simulink model "LoFT_Example3"  (R2024b)
settings: Solver=ode4  StartTime=0.0  StopTime=300  FixedStep=simu.dt  RelTol=1e-3
undefined symbols (not defined in the file): body, circtime, Communication, D1, Delta, irkb, line, LoFT, p0, Pn, s, simu, trip_time, Turbwind, waves, wind
libraries: simulink x350, spsThreePhaseVIMeasurementLib x41, spsThreePhasePISectionLineLib x34, spsThreePhaseParallelRLCLoadLib x21, spsThreePhaseTransformerTwoWindingsLib x14, spsLoadFlowBusLib x10, spsThreePhaseDynamicLoadLib x9, spsSynchronousMachinepuStandardLib x7, spsExcitationSystemLib x7, spsSteamTurbineandGovernorLib x7, spsGenericPowerSystemStabilizerLib x7, spsMultiBandPowerSystemStabilizerLib x7
(part 9 of 49)

== system LoFT_Example3/FOWT System/Subsystem5/wave series 2 ==
  1-D Lookup Table : Lookup_n-D  NumberOfTableDimensions=1  BreakpointsForDimension1=LoFT.Hydro.waveforces.time + 5  Table=squeeze(LoFT.Hydro.waveforces.force(1,1,:))  InternalRulePriority=Speed  RndMeth=Simplest
  1-D Lookup Table1 : Lookup_n-D  NumberOfTableDimensions=1  BreakpointsForDimension1=LoFT.Hydro.waveforces.time + 5  Table=squeeze(LoFT.Hydro.waveforces.force(1,2,:))  InternalRulePriority=Speed  RndMeth=Simplest
  1-D Lookup Table2 : Lookup_n-D  NumberOfTableDimensions=1  BreakpointsForDimension1=LoFT.Hydro.waveforces.time + 5  Table=squeeze(LoFT.Hydro.waveforces.force(1,3,:))  InternalRulePriority=Speed  RndMeth=Simplest
  Clock1 : Clock
  Clock2 : Clock
  Clock3 : Clock
  Vector Concatenate1 : Concatenate  NumInputs=3
  Out1 : Outport
  wires:
  Vector Concatenate1/1 -> Out1/1
  Clock2/1 -> 1-D Lookup Table1/1
  1-D Lookup Table/1 -> Vector Concatenate1/1
  Clock3/1 -> 1-D Lookup Table2/1
  Clock1/1 -> 1-D Lookup Table/1
  1-D Lookup Table1/1 -> Vector Concatenate1/2
  1-D Lookup Table2/1 -> Vector Concatenate1/3

== system LoFT_Example3/FOWT System/Subsystem5/wave series 3 ==
  1-D Lookup Table : Lookup_n-D  NumberOfTableDimensions=1  BreakpointsForDimension1=LoFT.Hydro.waveforces.time + 10  Table=squeeze(LoFT.Hydro.waveforces.force(1,1,:))  InternalRulePriority=Speed  RndMeth=Simplest
  1-D Lookup Table1 : Lookup_n-D  NumberOfTableDimensions=1  BreakpointsForDimension1=LoFT.Hydro.waveforces.time + 10  Table=squeeze(LoFT.Hydro.waveforces.force(1,2,:))  InternalRulePriority=Speed  RndMeth=Simplest
  1-D Lookup Table2 : Lookup_n-D  NumberOfTableDimensions=1  BreakpointsForDimension1=LoFT.Hydro.waveforces.time + 10  Table=squeeze(LoFT.Hydro.waveforces.force(1,3,:))  InternalRulePriority=Speed  RndMeth=Simplest
  Clock1 : Clock
  Clock2 : Clock
  Clock3 : Clock
  Vector Concatenate1 : Concatenate  NumInputs=3
  Out1 : Outport
  wires:
  1-D Lookup Table2/1 -> Vector Concatenate1/3
  1-D Lookup Table1/1 -> Vector Concatenate1/2
  Clock1/1 -> 1-D Lookup Table/1
  Clock3/1 -> 1-D Lookup Table2/1
  1-D Lookup Table/1 -> Vector Concatenate1/1
  Clock2/1 -> 1-D Lookup Table1/1
  Vector Concatenate1/1 -> Out1/1

== system LoFT_Example3/FOWT System/Subsystem5/wave series 4 ==
  1-D Lookup Table : Lookup_n-D  NumberOfTableDimensions=1  BreakpointsForDimension1=LoFT.Hydro.waveforces.time+15  Table=squeeze(LoFT.Hydro.waveforces.force(1,1,:))  InternalRulePriority=Speed  RndMeth=Simplest
  1-D Lookup Table1 : Lookup_n-D  NumberOfTableDimensions=1  BreakpointsForDimension1=LoFT.Hydro.waveforces.time+15  Table=squeeze(LoFT.Hydro.waveforces.force(1,2,:))  InternalRulePriority=Speed  RndMeth=Simplest
  1-D Lookup Table2 : Lookup_n-D  NumberOfTableDimensions=1  BreakpointsForDimension1=LoFT.Hydro.waveforces.time+15  Table=squeeze(LoFT.Hydro.waveforces.force(1,3,:))  InternalRulePriority=Speed  RndMeth=Simplest
  Clock1 : Clock
  Clock2 : Clock
  Clock3 : Clock
  Vector Concatenate1 : Concatenate  NumInputs=3
  Out1 : Outport
  wires:
  Vector Concatenate1/1 -> Out1/1
  Clock2/1 -> 1-D Lookup Table1/1
  1-D Lookup Table/1 -> Vector Concatenate1/1
  Clock3/1 -> 1-D Lookup Table2/1
  Clock1/1 -> 1-D Lookup Table/1
  1-D Lookup Table1/1 -> Vector Concatenate1/2
  1-D Lookup Table2/1 -> Vector Concatenate1/3

== system LoFT_Example3/FOWT System/Subsystem5/wave series 5 ==
  1-D Lookup Table : Lookup_n-D  NumberOfTableDimensions=1  BreakpointsForDimension1=LoFT.Hydro.waveforces.time+20  Table=squeeze(LoFT.Hydro.waveforces.force(1,1,:))  InternalRulePriority=Speed  RndMeth=Simplest
  1-D Lookup Table1 : Lookup_n-D  NumberOfTableDimensions=1  BreakpointsForDimension1=LoFT.Hydro.waveforces.time+20  Table=squeeze(LoFT.Hydro.waveforces.force(1,2,:))  InternalRulePriority=Speed  RndMeth=Simplest
  1-D Lookup Table2 : Lookup_n-D  NumberOfTableDimensions=1  BreakpointsForDimension1=LoFT.Hydro.waveforces.time+20  Table=squeeze(LoFT.Hydro.waveforces.force(1,3,:))  InternalRulePriority=Speed  RndMeth=Simplest
  Clock1 : Clock
  Clock2 : Clock
  Clock3 : Clock
  Vector Concatenate1 : Concatenate  NumInputs=3
  Out1 : Outport
  wires:
  1-D Lookup Table2/1 -> Vector Concatenate1/3
  1-D Lookup Table1/1 -> Vector Concatenate1/2
  Clock1/1 -> 1-D Lookup Table/1
  Clock3/1 -> 1-D Lookup Table2/1
  1-D Lookup Table/1 -> Vector Concatenate1/1
  Clock2/1 -> 1-D Lookup Table1/1
  Vector Concatenate1/1 -> Out1/1

== system LoFT_Example3/FOWT System/Subsystem5/wave series 6 ==
  1-D Lookup Table : Lookup_n-D  NumberOfTableDimensions=1  BreakpointsForDimension1=LoFT.Hydro.waveforces.time + 10  Table=squeeze(LoFT.Hydro.waveforces.force(1,1,:))  InternalRulePriority=Speed  RndMeth=Simplest
  1-D Lookup Table1 : Lookup_n-D  NumberOfTableDimensions=1  BreakpointsForDimension1=LoFT.Hydro.waveforces.time + 10  Table=squeeze(LoFT.Hydro.waveforces.force(1,2,:))  InternalRulePriority=Speed  RndMeth=Simplest
  1-D Lookup Table2 : Lookup_n-D  NumberOfTableDimensions=1  BreakpointsForDimension1=LoFT.Hydro.waveforces.time + 10  Table=squeeze(LoFT.Hydro.waveforces.force(1,3,:))  InternalRulePriority=Speed  RndMeth=Simplest
  Clock1 : Clock
  Clock2 : Clock
  Clock3 : Clock
  Vector Concatenate1 : Concatenate  NumInputs=3
  Out1 : Outport
  wires:
  Vector Concatenate1/1 -> Out1/1
  Clock2/1 -> 1-D Lookup Table1/1
  1-D Lookup Table/1 -> Vector Concatenate1/1
  Clock3/1 -> 1-D Lookup Table2/1
  Clock1/1 -> 1-D Lookup Table/1
  1-D Lookup Table1/1 -> Vector Concatenate1/2
  1-D Lookup Table2/1 -> Vector Concatenate1/3

== system LoFT_Example3/FOWT System/Subsystem5/wave series 7 ==
  1-D Lookup Table : Lookup_n-D  NumberOfTableDimensions=1  BreakpointsForDimension1=LoFT.Hydro.waveforces.time + 10  Table=squeeze(LoFT.Hydro.waveforces.force(1,1,:))  InternalRulePriority=Speed  RndMeth=Simplest
  1-D Lookup Table1 : Lookup_n-D  NumberOfTableDimensions=1  BreakpointsForDimension1=LoFT.Hydro.waveforces.time + 10  Table=squeeze(LoFT.Hydro.waveforces.force(1,2,:))  InternalRulePriority=Speed  RndMeth=Simplest
  1-D Lookup Table2 : Lookup_n-D  NumberOfTableDimensions=1  BreakpointsForDimension1=LoFT.Hydro.waveforces.time + 10  Table=squeeze(LoFT.Hydro.waveforces.force(1,3,:))  InternalRulePriority=Speed  RndMeth=Simplest
  Clock1 : Clock
  Clock2 : Clock
  Clock3 : Clock
  Vector Concatenate1 : Concatenate  NumInputs=3
  Out1 : Outport
  wires:
  1-D Lookup Table2/1 -> Vector Concatenate1/3
  1-D Lookup Table1/1 -> Vector Concatenate1/2
  Clock1/1 -> 1-D Lookup Table/1
  Clock3/1 -> 1-D Lookup Table2/1
  1-D Lookup Table/1 -> Vector Concatenate1/1
  Clock2/1 -> 1-D Lookup Table1/1
  Vector Concatenate1/1 -> Out1/1

== system LoFT_Example3/FOWT System/Subsystem5/wave series 8 ==
  1-D Lookup Table : Lookup_n-D  NumberOfTableDimensions=1  BreakpointsForDimension1=LoFT.Hydro.waveforces.time + 10  Table=squeeze(LoFT.Hydro.waveforces.force(1,1,:))  InternalRulePriority=Speed  RndMeth=Simplest
  1-D Lookup Table1 : Lookup_n-D  NumberOfTableDimensions=1  BreakpointsForDimension1=LoFT.Hydro.waveforces.time + 10  Table=squeeze(LoFT.Hydro.waveforces.force(1,2,:))  InternalRulePriority=Speed  RndMeth=Simplest
  1-D Lookup Table2 : Lookup_n-D  NumberOfTableDimensions=1  BreakpointsForDimension1=LoFT.Hydro.waveforces.time + 10  Table=squeeze(LoFT.Hydro.waveforces.force(1,3,:))  InternalRulePriority=Speed  RndMeth=Simplest
  Clock1 : Clock
  Clock2 : Clock
  Clock3 : Clock
  Vector Concatenate1 : Concatenate  NumInputs=3
  Out1 : Outport
  wires:
  Vector Concatenate1/1 -> Out1/1
  Clock2/1 -> 1-D Lookup Table1/1
  1-D Lookup Table/1 -> Vector Concatenate1/1
  Clock3/1 -> 1-D Lookup Table2/1
  Clock1/1 -> 1-D Lookup Table/1
  1-D Lookup Table1/1 -> Vector Concatenate1/2
  1-D Lookup Table2/1 -> Vector Concatenate1/3

== system LoFT_Example3/FOWT System/Subsystem5/wave series 9 ==
  1-D Lookup Table : Lookup_n-D  NumberOfTableDimensions=1  BreakpointsForDimension1=LoFT.Hydro.waveforces.time + 10  Table=squeeze(LoFT.Hydro.waveforces.force(1,1,:))  InternalRulePriority=Speed  RndMeth=Simplest
  1-D Lookup Table1 : Lookup_n-D  NumberOfTableDimensions=1  BreakpointsForDimension1=LoFT.Hydro.waveforces.time + 10  Table=squeeze(LoFT.Hydro.waveforces.force(1,2,:))  InternalRulePriority=Speed  RndMeth=Simplest
  1-D Lookup Table2 : Lookup_n-D  NumberOfTableDimensions=1  BreakpointsForDimension1=LoFT.Hydro.waveforces.time + 10  Table=squeeze(LoFT.Hydro.waveforces.force(1,3,:))  InternalRulePriority=Speed  RndMeth=Simplest
  Clock1 : Clock
  Clock2 : Clock
  Clock3 : Clock
  Vector Concatenate1 : Concatenate  NumInputs=3
  Out1 : Outport
  wires:
  Vector Concatenate1/1 -> Out1/1
  Clock2/1 -> 1-D Lookup Table1/1
  1-D Lookup Table/1 -> Vector Concatenate1/1
  Clock3/1 -> 1-D Lookup Table2/1
  Clock1/1 -> 1-D Lookup Table/1
  1-D Lookup Table1/1 -> Vector Concatenate1/2
  1-D Lookup Table2/1 -> Vector Concatenate1/3

== system LoFT_Example3/FOWT System/Subsystem7/FOWT1 ==
  Inflow wind(m/s) : Inport
  Waveforces : Inport  Port=2
  Power(MW) : Inport  Port=3
  Blade Pitch(rad) : Inport  Port=4
  Commu : Inport  Port=5
  3dof (Body Axes) : EOM3DOF  v_ini=0.01  theta_ini=Initposition(3)  pos_ini=[Initposition(1) Initposition(2)]  mass=Property.masstot  Iyy=Property.pitchinertia  g_in=External
  Add : Sum  Inputs=+-++
  Aerodynamics and Local Control Systems : Subsystem
  Constant : Constant  Value=0
  Delay : Delay  DelayLength=1  InitialCondition=0
  Delay1 : Delay  DelayLength=1  InitialCondition=0
  Delay2 : Delay  DelayLength=1  InitialCondition=0
  Demux : Demux  Outputs=3
  Gain : Gain  Gain=1e6
  Hydrodynamics : Subsystem
  Hydrostatics : Subsystem
  Measurements : Subsystem
  Moorings : Subsystem
  Subsystem1 : Subsystem
  wind speed(m/s) : Subsystem
  Out1 : Outport
  wires:
  Blade Pitch(rad)/1 -> Aerodynamics and Local Control Systems/5(Blade Pitch)
  wind speed(m/s)/2(Measured) -> Aerodynamics and Local Control Systems/2("Measureed ")
  [Acceleration] -> Hydrodynamics/1(Acceleration)
  Delay/1 -> [Position]
  Delay2/1 -> [Speed]
  Delay1/1 -> [Acceleration]
  Inflow wind(m/s)/1 -> wind speed(m/s)/1(Inflow)
  Subsystem1/4(Out3) -> Delay1/1
  Subsystem1/3(Out2) -> Delay2/1
  Gain/1 -> Aerodynamics and Local Control Systems/4(Power)
  Subsystem1/2(Out1) -> Delay/1
  wind speed(m/s)/1(Effective) -> Aerodynamics and Local Control Systems/1(WindSpeed)
  [Position] -> Moorings/1(position), Hydrostatics/1(position)
  Hydrostatics/1(Out1) -> Add/2  "F_hydrostatic"
  Constant/1 -> 3dof (Body Axes)/4
  Moorings/1(Out1) -> Add/3  "F_mooring"
  3dof (Body Axes)/1 -> Subsystem1/1(In1)
  3dof (Body Axes)/2 -> Subsystem1/2(In2)
  3dof (Body Axes)/3 -> Subsystem1/3(In3)
  3dof (Body Axes)/4 -> Subsystem1/4(In4)
  3dof (Body Axes)/5 -> Subsystem1/5(In5)
  3dof (Body Axes)/6 -> Subsystem1/6(In6)
  Add/1 -> Demux/1
  Demux/1 -> 3dof (Body Axes)/1
  Demux/2 -> 3dof (Body Axes)/2
  Demux/3 -> 3dof (Body Axes)/3
  [Speed] -> Hydrodynamics/2(Speed)
  Hydrodynamics/1(Out1) -> Add/4  "F_hydrodynamic"
  [Position] -> Hydrodynamics/3(Position)
  [Speed] -> wind speed(m/s)/2(In2)
  Aerodynamics and Local Control Systems/3(F_aero) -> Add/1
  Commu/1 -> Aerodynamics and Local Control Systems/6(Switch)
  Waveforces/1 -> Hydrodynamics/4(Wave)
  Subsystem1/1(Out4) -> Measurements/3(platform)
  Aerodynamics and Local Control Systems/1(Nacelle) -> Measurements/1(Nacelle)
  Measurements/1(Out1) -> Out1/1
  Aerodynamics and Local Control Systems/2(drivetrain) -> Measurements/2(drivetrain)
  wind speed(m/s)/3(FB) -> Aerodynamics and Local Control Systems/3(Nacelle Speed)
  Power(MW)/1 -> Gain/1

== system LoFT_Example3/FOWT System/Subsystem7/FOWT10 ==
  Inflow wind(m/s) : Inport
  Waveforces : Inport  Port=2
  Power(MW) : Inport  Port=3
  Blade Pitch(rad) : Inport  Port=4
  Commu : Inport  Port=5
  3dof (Body Axes) : EOM3DOF  v_ini=0.01  theta_ini=Initposition(3)  pos_ini=[Initposition(1) Initposition(2)]  mass=Property.masstot  Iyy=Property.pitchinertia  g_in=External
  Add : Sum  Inputs=+-++
  Aerodynamics and Local Control Systems : Subsystem
  Constant : Constant  Value=0
  Delay : Delay  DelayLength=1  InitialCondition=0
  Delay1 : Delay  DelayLength=1  InitialCondition=0
  Delay2 : Delay  DelayLength=1  InitialCondition=0
  Demux : Demux  Outputs=3
  Gain : Gain  Gain=1e6
  Hydrodynamics : Subsystem
  Hydrostatics : Subsystem
  Measurements : Subsystem
  Moorings : Subsystem
  Subsystem1 : Subsystem
  wind speed(m/s) : Subsystem
  Out1 : Outport
  wires:
  Power(MW)/1 -> Gain/1
  wind speed(m/s)/3(FB) -> Aerodynamics and Local Control Systems/3(Nacelle Speed)
  Aerodynamics and Local Control Systems/2(drivetrain) -> Measurements/2(drivetrain)
  Measurements/1(Out1) -> Out1/1
  Aerodynamics and Local Control Systems/1(Nacelle) -> Measurements/1(Nacelle)
  Subsystem1/1(Out4) -> Measurements/3(platform)
  Waveforces/1 -> Hydrodynamics/4(Wave)
  Commu/1 -> Aerodynamics and Local Control Systems/6(Switch)
  Aerodynamics and Local Control Systems/3(F_aero) -> Add/1
  [Speed] -> wind speed(m/s)/2(In2)
  [Position] -> Hydrodynamics/3(Position)
  Hydrodynamics/1(Out1) -> Add/4  "F_hydrodynamic"
  [Speed] -> Hydrodynamics/2(Speed)
  Demux/3 -> 3dof (Body Axes)/3
  Demux/2 -> 3dof (Body Axes)/2
  Demux/1 -> 3dof (Body Axes)/1
  Add/1 -> Demux/1
  3dof (Body Axes)/6 -> Subsystem1/6(In6)
  3dof (Body Axes)/5 -> Subsystem1/5(In5)
  3dof (Body Axes)/4 -> Subsystem1/4(In4)
  3dof (Body Axes)/3 -> Subsystem1/3(In3)
  3dof (Body Axes)/2 -> Subsystem1/2(In2)
  3dof (Body Axes)/1 -> Subsystem1/1(In1)
  Moorings/1(Out1) -> Add/3  "F_mooring"
  Constant/1 -> 3dof (Body Axes)/4
  Hydrostatics/1(Out1) -> Add/2  "F_hydrostatic"
  [Position] -> Hydrostatics/1(position), Moorings/1(position)
  wind speed(m/s)/1(Effective) -> Aerodynamics and Local Control Systems/1(WindSpeed)
  Subsystem1/2(Out1) -> Delay/1
  Gain/1 -> Aerodynamics and Local Control Systems/4(Power)
  Subsystem1/3(Out2) -> Delay2/1
  Subsystem1/4(Out3) -> Delay1/1
  Inflow wind(m/s)/1 -> wind speed(m/s)/1(Inflow)
  Delay1/1 -> [Acceleration]
  Delay2/1 -> [Speed]
  Delay/1 -> [Position]
  [Acceleration] -> Hydrodynamics/1(Acceleration)
  wind speed(m/s)/2(Measured) -> Aerodynamics and Local Control Systems/2("Measureed ")
  Blade Pitch(rad)/1 -> Aerodynamics and Local Control Systems/5(Blade Pitch)

== system LoFT_Example3/FOWT System/Subsystem7/FOWT2 ==
  Inflow wind(m/s) : Inport
  Waveforces : Inport  Port=2
  Power(MW) : Inport  Port=3
  Blade Pitch(rad) : Inport  Port=4
  Commu : Inport  Port=5
  3dof (Body Axes) : EOM3DOF  v_ini=0.01  theta_ini=Initposition(3)  pos_ini=[Initposition(1) Initposition(2)]  mass=Property.masstot  Iyy=Property.pitchinertia  g_in=External
  Add : Sum  Inputs=+-++
  Aerodynamics and Local Control Systems : Subsystem
  Constant : Constant  Value=0
  Delay : Delay  DelayLength=1  InitialCondition=0
  Delay1 : Delay  DelayLength=1  InitialCondition=0
  Delay2 : Delay  DelayLength=1  InitialCondition=0
  Demux : Demux  Outputs=3
  Gain : Gain  Gain=1e6
  Hydrodynamics : Subsystem
  Hydrostatics : Subsystem
  Measurements : Subsystem
  Moorings : Subsystem
  Subsystem1 : Subsystem
  wind speed(m/s) : Subsystem
  Out1 : Outport
  wires:
  Power(MW)/1 -> Gain/1
  wind speed(m/s)/3(FB) -> Aerodynamics and Local Control Systems/3(Nacelle Speed)
  Aerodynamics and Local Control Systems/2(drivetrain) -> Measurements/2(drivetrain)
  Measurements/1(Out1) -> Out1/1
  Aerodynamics and Local Control Systems/1(Nacelle) -> Measurements/1(Nacelle)
  Subsystem1/1(Out4) -> Measurements/3(platform)
  Waveforces/1 -> Hydrodynamics/4(Wave)
  Commu/1 -> Aerodynamics and Local Control Systems/6(Switch)
  Aerodynamics and Local Control Systems/3(F_aero) -> Add/1
  [Speed] -> wind speed(m/s)/2(In2)
  [Position] -> Hydrodynamics/3(Position)
  Hydrodynamics/1(Out1) -> Add/4  "F_hydrodynamic"
  [Speed] -> Hydrodynamics/2(Speed)
  Demux/3 -> 3dof (Body Axes)/3
  Demux/2 -> 3dof (Body Axes)/2
  Demux/1 -> 3dof (Body Axes)/1
  Add/1 -> Demux/1
  3dof (Body Axes)/6 -> Subsystem1/6(In6)
  3dof (Body Axes)/5 -> Subsystem1/5(In5)
  3dof (Body Axes)/4 -> Subsystem1/4(In4)
  3dof (Body Axes)/3 -> Subsystem1/3(In3)
  3dof (Body Axes)/2 -> Subsystem1/2(In2)
  3dof (Body Axes)/1 -> Subsystem1/1(In1)
  Moorings/1(Out1) -> Add/3  "F_mooring"
  Constant/1 -> 3dof (Body Axes)/4
  Hydrostatics/1(Out1) -> Add/2  "F_hydrostatic"
  [Position] -> Hydrostatics/1(position), Moorings/1(position)
  wind speed(m/s)/1(Effective) -> Aerodynamics and Local Control Systems/1(WindSpeed)
  Subsystem1/2(Out1) -> Delay/1
  Gain/1 -> Aerodynamics and Local Control Systems/4(Power)
  Subsystem1/3(Out2) -> Delay2/1
  Subsystem1/4(Out3) -> Delay1/1
  Inflow wind(m/s)/1 -> wind speed(m/s)/1(Inflow)
  Delay1/1 -> [Acceleration]
  Delay2/1 -> [Speed]
  Delay/1 -> [Position]
  [Acceleration] -> Hydrodynamics/1(Acceleration)
  wind speed(m/s)/2(Measured) -> Aerodynamics and Local Control Systems/2("Measureed ")
  Blade Pitch(rad)/1 -> Aerodynamics and Local Control Systems/5(Blade Pitch)

== system LoFT_Example3/FOWT System/Subsystem7/FOWT3 ==
  Inflow wind(m/s) : Inport
  Waveforces : Inport  Port=2
  Power(MW) : Inport  Port=3
  Blade Pitch(rad) : Inport  Port=4
  Commu : Inport  Port=5
  3dof (Body Axes) : EOM3DOF  v_ini=0.01  theta_ini=Initposition(3)  pos_ini=[Initposition(1) Initposition(2)]  mass=Property.masstot  Iyy=Property.pitchinertia  g_in=External
  Add : Sum  Inputs=+-++
  Aerodynamics and Local Control Systems : Subsystem
  Constant : Constant  Value=0
  Delay : Delay  DelayLength=1  InitialCondition=0
  Delay1 : Delay  DelayLength=1  InitialCondition=0
  Delay2 : Delay  DelayLength=1  InitialCondition=0
  Demux : Demux  Outputs=3
  Gain : Gain  Gain=1e6
  Hydrodynamics : Subsystem
  Hydrostatics : Subsystem
  Measurements : Subsystem
  Moorings : Subsystem
  Subsystem1 : Subsystem
  wind speed(m/s) : Subsystem
  Out1 : Outport
  wires:
  Blade Pitch(rad)/1 -> Aerodynamics and Local Control Systems/5(Blade Pitch)
  wind speed(m/s)/2(Measured) -> Aerodynamics and Local Control Systems/2("Measureed ")
  [Acceleration] -> Hydrodynamics/1(Acceleration)
  Delay/1 -> [Position]
  Delay2/1 -> [Speed]
  Delay1/1 -> [Acceleration]
  Inflow wind(m/s)/1 -> wind speed(m/s)/1(Inflow)
  Subsystem1/4(Out3) -> Delay1/1
  Subsystem1/3(Out2) -> Delay2/1
  Gain/1 -> Aerodynamics and Local Control Systems/4(Power)
  Subsystem1/2(Out1) -> Delay/1
  wind speed(m/s)/1(Effective) -> Aerodynamics and Local Control Systems/1(WindSpeed)
  [Position] -> Moorings/1(position), Hydrostatics/1(position)
  Hydrostatics/1(Out1) -> Add/2  "F_hydrostatic"
  Constant/1 -> 3dof (Body Axes)/4
  Moorings/1(Out1) -> Add/3  "F_mooring"
  3dof (Body Axes)/1 -> Subsystem1/1(In1)
  3dof (Body Axes)/2 -> Subsystem1/2(In2)
  3dof (Body Axes)/3 -> Subsystem1/3(In3)
  3dof (Body Axes)/4 -> Subsystem1/4(In4)
  3dof (Body Axes)/5 -> Subsystem1/5(In5)
  3dof (Body Axes)/6 -> Subsystem1/6(In6)
  Add/1 -> Demux/1
  Demux/1 -> 3dof (Body Axes)/1
  Demux/2 -> 3dof (Body Axes)/2
  Demux/3 -> 3dof (Body Axes)/3
  [Speed] -> Hydrodynamics/2(Speed)
  Hydrodynamics/1(Out1) -> Add/4  "F_hydrodynamic"
  [Position] -> Hydrodynamics/3(Position)
  [Speed] -> wind speed(m/s)/2(In2)
  Aerodynamics and Local Control Systems/3(F_aero) -> Add/1
  Commu/1 -> Aerodynamics and Local Control Systems/6(Switch)
  Waveforces/1 -> Hydrodynamics/4(Wave)
  Subsystem1/1(Out4) -> Measurements/3(platform)
  Aerodynamics and Local Control Systems/1(Nacelle) -> Measurements/1(Nacelle)
  Measurements/1(Out1) -> Out1/1
  Aerodynamics and Local Control Systems/2(drivetrain) -> Measurements/2(drivetrain)
  wind speed(m/s)/3(FB) -> Aerodynamics and Local Control Systems/3(Nacelle Speed)
  Power(MW)/1 -> Gain/1

== system LoFT_Example3/FOWT System/Subsystem7/FOWT4 ==
  Inflow wind(m/s) : Inport
  Waveforces : Inport  Port=2
  Power(MW) : Inport  Port=3
  Blade Pitch(rad) : Inport  Port=4
  Commu : Inport  Port=5
  3dof (Body Axes) : EOM3DOF  v_ini=0.01  theta_ini=Initposition(3)  pos_ini=[Initposition(1) Initposition(2)]  mass=Property.masstot  Iyy=Property.pitchinertia  g_in=External
  Add : Sum  Inputs=+-++
  Aerodynamics and Local Control Systems : Subsystem
  Constant : Constant  Value=0
  Delay : Delay  DelayLength=1  InitialCondition=0
  Delay1 : Delay  DelayLength=1  InitialCondition=0
  Delay2 : Delay  DelayLength=1  InitialCondition=0
  Demux : Demux  Outputs=3
  Gain : Gain  Gain=1e6
  Hydrodynamics : Subsystem
  Hydrostatics : Subsystem
  Measurements : Subsystem
  Moorings : Subsystem
  Subsystem1 : Subsystem
  wind speed(m/s) : Subsystem
  Out1 : Outport
  wires:
  Power(MW)/1 -> Gain/1
  wind speed(m/s)/3(FB) -> Aerodynamics and Local Control Systems/3(Nacelle Speed)
  Aerodynamics and Local Control Systems/2(drivetrain) -> Measurements/2(drivetrain)
  Measurements/1(Out1) -> Out1/1
  Aerodynamics and Local Control Systems/1(Nacelle) -> Measurements/1(Nacelle)
  Subsystem1/1(Out4) -> Measurements/3(platform)
  Waveforces/1 -> Hydrodynamics/4(Wave)
  Commu/1 -> Aerodynamics and Local Control Systems/6(Switch)
  Aerodynamics and Local Control Systems/3(F_aero) -> Add/1
  [Speed] -> wind speed(m/s)/2(In2)
  [Position] -> Hydrodynamics/3(Position)
  Hydrodynamics/1(Out1) -> Add/4  "F_hydrodynamic"
  [Speed] -> Hydrodynamics/2(Speed)
  Demux/3 -> 3dof (Body Axes)/3
  Demux/2 -> 3dof (Body Axes)/2
  Demux/1 -> 3dof (Body Axes)/1
  Add/1 -> Demux/1
  3dof (Body Axes)/6 -> Subsystem1/6(In6)
  3dof (Body Axes)/5 -> Subsystem1/5(In5)
  3dof (Body Axes)/4 -> Subsystem1/4(In4)
  3dof (Body Axes)/3 -> Subsystem1/3(In3)
  3dof (Body Axes)/2 -> Subsystem1/2(In2)
  3dof (Body Axes)/1 -> Subsystem1/1(In1)
  Moorings/1(Out1) -> Add/3  "F_mooring"
  Constant/1 -> 3dof (Body Axes)/4
  Hydrostatics/1(Out1) -> Add/2  "F_hydrostatic"
  [Position] -> Hydrostatics/1(position), Moorings/1(position)
  wind speed(m/s)/1(Effective) -> Aerodynamics and Local Control Systems/1(WindSpeed)
  Subsystem1/2(Out1) -> Delay/1
  Gain/1 -> Aerodynamics and Local Control Systems/4(Power)
  Subsystem1/3(Out2) -> Delay2/1
  Subsystem1/4(Out3) -> Delay1/1
  Inflow wind(m/s)/1 -> wind speed(m/s)/1(Inflow)
  Delay1/1 -> [Acceleration]
  Delay2/1 -> [Speed]
  Delay/1 -> [Position]
  [Acceleration] -> Hydrodynamics/1(Acceleration)
  wind speed(m/s)/2(Measured) -> Aerodynamics and Local Control Systems/2("Measureed ")
  Blade Pitch(rad)/1 -> Aerodynamics and Local Control Systems/5(Blade Pitch)

== system LoFT_Example3/FOWT System/Subsystem7/FOWT5 ==
  Inflow wind(m/s) : Inport
  Waveforces : Inport  Port=2
  Power(MW) : Inport  Port=3
  Blade Pitch(rad) : Inport  Port=4
  Commu : Inport  Port=5
  3dof (Body Axes) : EOM3DOF  v_ini=0.01  theta_ini=Initposition(3)  pos_ini=[Initposition(1) Initposition(2)]  mass=Property.masstot  Iyy=Property.pitchinertia  g_in=External
  Add : Sum  Inputs=+-++
  Aerodynamics and Local Control Systems : Subsystem
  Constant : Constant  Value=0
  Delay : Delay  DelayLength=1  InitialCondition=0
  Delay1 : Delay  DelayLength=1  InitialCondition=0
  Delay2 : Delay  DelayLength=1  InitialCondition=0
  Demux : Demux  Outputs=3
  Gain : Gain  Gain=1e6
  Hydrodynamics : Subsystem
  Hydrostatics : Subsystem
  Measurements : Subsystem
  Moorings : Subsystem
  Subsystem1 : Subsystem
  wind speed(m/s) : Subsystem
  Out1 : Outport
  wires:
  Blade Pitch(rad)/1 -> Aerodynamics and Local Control Systems/5(Blade Pitch)
  wind speed(m/s)/2(Measured) -> Aerodynamics and Local Control Systems/2("Measureed ")
  [Acceleration] -> Hydrodynamics/1(Acceleration)
  Delay/1 -> [Position]
  Delay2/1 -> [Speed]
  Delay1/1 -> [Acceleration]
  Inflow wind(m/s)/1 -> wind speed(m/s)/1(Inflow)
  Subsystem1/4(Out3) -> Delay1/1
  Subsystem1/3(Out2) -> Delay2/1
  Gain/1 -> Aerodynamics and Local Control Systems/4(Power)
  Subsystem1/2(Out1) -> Delay/1
  wind speed(m/s)/1(Effective) -> Aerodynamics and Local Control Systems/1(WindSpeed)
  [Position] -> Moorings/1(position), Hydrostatics/1(position)
  Hydrostatics/1(Out1) -> Add/2  "F_hydrostatic"
  Constant/1 -> 3dof (Body Axes)/4
  Moorings/1(Out1) -> Add/3  "F_mooring"
  3dof (Body Axes)/1 -> Subsystem1/1(In1)
  3dof (Body Axes)/2 -> Subsystem1/2(In2)
  3dof (Body Axes)/3 -> Subsystem1/3(In3)
  3dof (Body Axes)/4 -> Subsystem1/4(In4)
  3dof (Body Axes)/5 -> Subsystem1/5(In5)
  3dof (Body Axes)/6 -> Subsystem1/6(In6)
  Add/1 -> Demux/1
  Demux/1 -> 3dof (Body Axes)/1
  Demux/2 -> 3dof (Body Axes)/2
  Demux/3 -> 3dof (Body Axes)/3
  [Speed] -> Hydrodynamics/2(Speed)
  Hydrodynamics/1(Out1) -> Add/4  "F_hydrodynamic"
  [Position] -> Hydrodynamics/3(Position)
  [Speed] -> wind speed(m/s)/2(In2)
  Aerodynamics and Local Control Systems/3(F_aero) -> Add/1
  Commu/1 -> Aerodynamics and Local Control Systems/6(Switch)
  Waveforces/1 -> Hydrodynamics/4(Wave)
  Subsystem1/1(Out4) -> Measurements/3(platform)
  Aerodynamics and Local Control Systems/1(Nacelle) -> Measurements/1(Nacelle)
  Measurements/1(Out1) -> Out1/1
  Aerodynamics and Local Control Systems/2(drivetrain) -> Measurements/2(drivetrain)
  wind speed(m/s)/3(FB) -> Aerodynamics and Local Control Systems/3(Nacelle Speed)
  Power(MW)/1 -> Gain/1

== system LoFT_Example3/FOWT System/Subsystem7/FOWT6 ==
  Inflow wind(m/s) : Inport
  Waveforces : Inport  Port=2
  Power(MW) : Inport  Port=3
  Blade Pitch(rad) : Inport  Port=4
  Commu : Inport  Port=5
  3dof (Body Axes) : EOM3DOF  v_ini=0.01  theta_ini=Initposition(3)  pos_ini=[Initposition(1) Initposition(2)]  mass=Property.masstot  Iyy=Property.pitchinertia  g_in=External
  Add : Sum  Inputs=+-++
  Aerodynamics and Local Control Systems : Subsystem
  Constant : Constant  Value=0
  Delay : Delay  DelayLength=1  InitialCondition=0
  Delay1 : Delay  DelayLength=1  InitialCondition=0
  Delay2 : Delay  DelayLength=1  InitialCondition=0
  Demux : Demux  Outputs=3
  Gain : Gain  Gain=1e6
  Hydrodynamics : Subsystem
  Hydrostatics : Subsystem
  Measurements : Subsystem
  Moorings : Subsystem
  Subsystem1 : Subsystem
  wind speed(m/s) : Subsystem
  Out1 : Outport
  wires:
  Power(MW)/1 -> Gain/1
  wind speed(m/s)/3(FB) -> Aerodynamics and Local Control Systems/3(Nacelle Speed)
  Aerodynamics and Local Control Systems/2(drivetrain) -> Measurements/2(drivetrain)
  Measurements/1(Out1) -> Out1/1
  Aerodynamics and Local Control Systems/1(Nacelle) -> Measurements/1(Nacelle)
  Subsystem1/1(Out4) -> Measurements/3(platform)
  Waveforces/1 -> Hydrodynamics/4(Wave)
  Commu/1 -> Aerodynamics and Local Control Systems/6(Switch)
  Aerodynamics and Local Control Systems/3(F_aero) -> Add/1
  [Speed] -> wind speed(m/s)/2(In2)
  [Position] -> Hydrodynamics/3(Position)
  Hydrodynamics/1(Out1) -> Add/4  "F_hydrodynamic"
  [Speed] -> Hydrodynamics/2(Speed)
  Demux/3 -> 3dof (Body Axes)/3
  Demux/2 -> 3dof (Body Axes)/2
  Demux/1 -> 3dof (Body Axes)/1
  Add/1 -> Demux/1
  3dof (Body Axes)/6 -> Subsystem1/6(In6)
  3dof (Body Axes)/5 -> Subsystem1/5(In5)
  3dof (Body Axes)/4 -> Subsystem1/4(In4)
  3dof (Body Axes)/3 -> Subsystem1/3(In3)
  3dof (Body Axes)/2 -> Subsystem1/2(In2)
  3dof (Body Axes)/1 -> Subsystem1/1(In1)
  Moorings/1(Out1) -> Add/3  "F_mooring"
  Constant/1 -> 3dof (Body Axes)/4
  Hydrostatics/1(Out1) -> Add/2  "F_hydrostatic"
  [Position] -> Hydrostatics/1(position), Moorings/1(position)
  wind speed(m/s)/1(Effective) -> Aerodynamics and Local Control Systems/1(WindSpeed)
  Subsystem1/2(Out1) -> Delay/1
  Gain/1 -> Aerodynamics and Local Control Systems/4(Power)
  Subsystem1/3(Out2) -> Delay2/1
  Subsystem1/4(Out3) -> Delay1/1
  Inflow wind(m/s)/1 -> wind speed(m/s)/1(Inflow)
  Delay1/1 -> [Acceleration]
  Delay2/1 -> [Speed]
  Delay/1 -> [Position]
  [Acceleration] -> Hydrodynamics/1(Acceleration)
  wind speed(m/s)/2(Measured) -> Aerodynamics and Local Control Systems/2("Measureed ")
  Blade Pitch(rad)/1 -> Aerodynamics and Local Control Systems/5(Blade Pitch)

== system LoFT_Example3/FOWT System/Subsystem7/FOWT7 ==
  Inflow wind(m/s) : Inport
  Waveforces : Inport  Port=2
  Power(MW) : Inport  Port=3
  Blade Pitch(rad) : Inport  Port=4
  Commu : Inport  Port=5
  3dof (Body Axes) : EOM3DOF  v_ini=0.01  theta_ini=Initposition(3)  pos_ini=[Initposition(1) Initposition(2)]  mass=Property.masstot  Iyy=Property.pitchinertia  g_in=External
  Add : Sum  Inputs=+-++
  Aerodynamics and Local Control Systems : Subsystem
  Constant : Constant  Value=0
  Delay : Delay  DelayLength=1  InitialCondition=0
  Delay1 : Delay  DelayLength=1  InitialCondition=0
  Delay2 : Delay  DelayLength=1  InitialCondition=0
  Demux : Demux  Outputs=3
  Gain : Gain  Gain=1e6
  Hydrodynamics : Subsystem
  Hydrostatics : Subsystem
  Measurements : Subsystem
  Moorings : Subsystem
  Subsystem1 : Subsystem
  wind speed(m/s) : Subsystem
  Out1 : Outport
  wires:
  Blade Pitch(rad)/1 -> Aerodynamics and Local Control Systems/5(Blade Pitch)
  wind speed(m/s)/2(Measured) -> Aerodynamics and Local Control Systems/2("Measureed ")
  [Acceleration] -> Hydrodynamics/1(Acceleration)
  Delay/1 -> [Position]
  Delay2/1 -> [Speed]
  Delay1/1 -> [Acceleration]
  Inflow wind(m/s)/1 -> wind speed(m/s)/1(Inflow)
  Subsystem1/4(Out3) -> Delay1/1
  Subsystem1/3(Out2) -> Delay2/1
  Gain/1 -> Aerodynamics and Local Control Systems/4(Power)
  Subsystem1/2(Out1) -> Delay/1
  wind speed(m/s)/1(Effective) -> Aerodynamics and Local Control Systems/1(WindSpeed)
  [Position] -> Moorings/1(position), Hydrostatics/1(position)
  Hydrostatics/1(Out1) -> Add/2  "F_hydrostatic"
  Constant/1 -> 3dof (Body Axes)/4
  Moorings/1(Out1) -> Add/3  "F_mooring"
  3dof (Body Axes)/1 -> Subsystem1/1(In1)
  3dof (Body Axes)/2 -> Subsystem1/2(In2)
  3dof (Body Axes)/3 -> Subsystem1/3(In3)
  3dof (Body Axes)/4 -> Subsystem1/4(In4)
  3dof (Body Axes)/5 -> Subsystem1/5(In5)
  3dof (Body Axes)/6 -> Subsystem1/6(In6)
  Add/1 -> Demux/1
  Demux/1 -> 3dof (Body Axes)/1
  Demux/2 -> 3dof (Body Axes)/2
  Demux/3 -> 3dof (Body Axes)/3
  [Speed] -> Hydrodynamics/2(Speed)
  Hydrodynamics/1(Out1) -> Add/4  "F_hydrodynamic"
  [Position] -> Hydrodynamics/3(Position)
  [Speed] -> wind speed(m/s)/2(In2)
  Aerodynamics and Local Control Systems/3(F_aero) -> Add/1
  Commu/1 -> Aerodynamics and Local Control Systems/6(Switch)
  Waveforces/1 -> Hydrodynamics/4(Wave)
  Subsystem1/1(Out4) -> Measurements/3(platform)
  Aerodynamics and Local Control Systems/1(Nacelle) -> Measurements/1(Nacelle)
  Measurements/1(Out1) -> Out1/1
  Aerodynamics and Local Control Systems/2(drivetrain) -> Measurements/2(drivetrain)
  wind speed(m/s)/3(FB) -> Aerodynamics and Local Control Systems/3(Nacelle Speed)
  Power(MW)/1 -> Gain/1

== system LoFT_Example3/FOWT System/Subsystem7/FOWT8 ==
  Inflow wind(m/s) : Inport
  Waveforces : Inport  Port=2
  Power(MW) : Inport  Port=3
  Blade Pitch(rad) : Inport  Port=4
  Commu : Inport  Port=5
  3dof (Body Axes) : EOM3DOF  v_ini=0.01  theta_ini=Initposition(3)  pos_ini=[Initposition(1) Initposition(2)]  mass=Property.masstot  Iyy=Property.pitchinertia  g_in=External
  Add : Sum  Inputs=+-++
  Aerodynamics and Local Control Systems : Subsystem
  Constant : Constant  Value=0
  Delay : Delay  DelayLength=1  InitialCondition=0
  Delay1 : Delay  DelayLength=1  InitialCondition=0
  Delay2 : Delay  DelayLength=1  InitialCondition=0
  Demux : Demux  Outputs=3
  Gain : Gain  Gain=1e6
  Hydrodynamics : Subsystem
  Hydrostatics : Subsystem
  Measurements : Subsystem
  Moorings : Subsystem
  Subsystem1 : Subsystem
  wind speed(m/s) : Subsystem
  Out1 : Outport
  wires:
  Power(MW)/1 -> Gain/1
  wind speed(m/s)/3(FB) -> Aerodynamics and Local Control Systems/3(Nacelle Speed)
  Aerodynamics and Local Control Systems/2(drivetrain) -> Measurements/2(drivetrain)
  Measurements/1(Out1) -> Out1/1
  Aerodynamics and Local Control Systems/1(Nacelle) -> Measurements/1(Nacelle)
  Subsystem1/1(Out4) -> Measurements/3(platform)
  Waveforces/1 -> Hydrodynamics/4(Wave)
  Commu/1 -> Aerodynamics and Local Control Systems/6(Switch)
  Aerodynamics and Local Control Systems/3(F_aero) -> Add/1
  [Speed] -> wind speed(m/s)/2(In2)
  [Position] -> Hydrodynamics/3(Position)
  Hydrodynamics/1(Out1) -> Add/4  "F_hydrodynamic"
  [Speed] -> Hydrodynamics/2(Speed)
  Demux/3 -> 3dof (Body Axes)/3
  Demux/2 -> 3dof (Body Axes)/2
  Demux/1 -> 3dof (Body Axes)/1
  Add/1 -> Demux/1
  3dof (Body Axes)/6 -> Subsystem1/6(In6)
  3dof (Body Axes)/5 -> Subsystem1/5(In5)
  3dof (Body Axes)/4 -> Subsystem1/4(In4)
  3dof (Body Axes)/3 -> Subsystem1/3(In3)
  3dof (Body Axes)/2 -> Subsystem1/2(In2)
  3dof (Body Axes)/1 -> Subsystem1/1(In1)
  Moorings/1(Out1) -> Add/3  "F_mooring"
  Constant/1 -> 3dof (Body Axes)/4
  Hydrostatics/1(Out1) -> Add/2  "F_hydrostatic"
  [Position] -> Hydrostatics/1(position), Moorings/1(position)
  wind speed(m/s)/1(Effective) -> Aerodynamics and Local Control Systems/1(WindSpeed)
  Subsystem1/2(Out1) -> Delay/1
  Gain/1 -> Aerodynamics and Local Control Systems/4(Power)
  Subsystem1/3(Out2) -> Delay2/1
  Subsystem1/4(Out3) -> Delay1/1
  Inflow wind(m/s)/1 -> wind speed(m/s)/1(Inflow)
  Delay1/1 -> [Acceleration]
  Delay2/1 -> [Speed]
  Delay/1 -> [Position]
  [Acceleration] -> Hydrodynamics/1(Acceleration)
  wind speed(m/s)/2(Measured) -> Aerodynamics and Local Control Systems/2("Measureed ")
  Blade Pitch(rad)/1 -> Aerodynamics and Local Control Systems/5(Blade Pitch)

== system LoFT_Example3/FOWT System/Subsystem7/FOWT9 ==
  Inflow wind(m/s) : Inport
  Waveforces : Inport  Port=2
  Power(MW) : Inport  Port=3
  Blade Pitch(rad) : Inport  Port=4
  Commu : Inport  Port=5
  3dof (Body Axes) : EOM3DOF  v_ini=0.01  theta_ini=Initposition(3)  pos_ini=[Initposition(1) Initposition(2)]  mass=Property.masstot  Iyy=Property.pitchinertia  g_in=External
  Add : Sum  Inputs=+-++
  Aerodynamics and Local Control Systems : Subsystem
  Constant : Constant  Value=0
  Delay : Delay  DelayLength=1  InitialCondition=0
  Delay1 : Delay  DelayLength=1  InitialCondition=0
  Delay2 : Delay  DelayLength=1  InitialCondition=0
  Demux : Demux  Outputs=3
  Gain : Gain  Gain=1e6
  Hydrodynamics : Subsystem
  Hydrostatics : Subsystem
  Measurements : Subsystem
  Moorings : Subsystem
  Subsystem1 : Subsystem
  wind speed(m/s) : Subsystem
  Out1 : Outport
  wires:
  Blade Pitch(rad)/1 -> Aerodynamics and Local Control Systems/5(Blade Pitch)
  wind speed(m/s)/2(Measured) -> Aerodynamics and Local Control Systems/2("Measureed ")
  [Acceleration] -> Hydrodynamics/1(Acceleration)
  Delay/1 -> [Position]
  Delay2/1 -> [Speed]
  Delay1/1 -> [Acceleration]
  Inflow wind(m/s)/1 -> wind speed(m/s)/1(Inflow)
  Subsystem1/4(Out3) -> Delay1/1
  Subsystem1/3(Out2) -> Delay2/1
  Gain/1 -> Aerodynamics and Local Control Systems/4(Power)
  Subsystem1/2(Out1) -> Delay/1
  wind speed(m/s)/1(Effective) -> Aerodynamics and Local Control Systems/1(WindSpeed)
  [Position] -> Moorings/1(position), Hydrostatics/1(position)
  Hydrostatics/1(Out1) -> Add/2  "F_hydrostatic"
  Constant/1 -> 3dof (Body Axes)/4
  Moorings/1(Out1) -> Add/3  "F_mooring"
  3dof (Body Axes)/1 -> Subsystem1/1(In1)
  3dof (Body Axes)/2 -> Subsystem1/2(In2)
  3dof (Body Axes)/3 -> Subsystem1/3(In3)
  3dof (Body Axes)/4 -> Subsystem1/4(In4)
  3dof (Body Axes)/5 -> Subsystem1/5(In5)
  3dof (Body Axes)/6 -> Subsystem1/6(In6)
  Add/1 -> Demux/1
  Demux/1 -> 3dof (Body Axes)/1
  Demux/2 -> 3dof (Body Axes)/2
  Demux/3 -> 3dof (Body Axes)/3
  [Speed] -> Hydrodynamics/2(Speed)
  Hydrodynamics/1(Out1) -> Add/4  "F_hydrodynamic"
  [Position] -> Hydrodynamics/3(Position)
  [Speed] -> wind speed(m/s)/2(In2)
  Aerodynamics and Local Control Systems/3(F_aero) -> Add/1
  Commu/1 -> Aerodynamics and Local Control Systems/6(Switch)
  Waveforces/1 -> Hydrodynamics/4(Wave)
  Subsystem1/1(Out4) -> Measurements/3(platform)
  Aerodynamics and Local Control Systems/1(Nacelle) -> Measurements/1(Nacelle)
  Measurements/1(Out1) -> Out1/1
  Aerodynamics and Local Control Systems/2(drivetrain) -> Measurements/2(drivetrain)
  wind speed(m/s)/3(FB) -> Aerodynamics and Local Control Systems/3(Nacelle Speed)
  Power(MW)/1 -> Gain/1

== system LoFT_Example3/FOWT System/Subsystem7/switch  ==
  note: communictation failure occurs when switch ==0
  In1 : Inport
  Constant : Constant  Value=0
  Mux : Mux  Inputs=2
  Out1 : Outport
  wires:
  Mux/1 -> Out1/1
  In1/1 -> Mux/1
  Constant/1 -> Mux/2

== system LoFT_Example3/FOWT System/Subsystem7/switch 1 ==
  note: communictation failure occurs when switch ==0
  In1 : Inport
  Constant : Constant  Value=0
  Mux : Mux  Inputs=2
  Out1 : Outport
  wires:
  Constant/1 -> Mux/2
  In1/1 -> Mux/1
  Mux/1 -> Out1/1

== system LoFT_Example3/FOWT System/Subsystem7/switch 2 ==
  note: communictation failure occurs when switch ==0
  In1 : Inport
  Constant : Constant  Value=0
  Mux : Mux  Inputs=2
  Out1 : Outport
  wires:
  Mux/1 -> Out1/1
  In1/1 -> Mux/1
  Constant/1 -> Mux/2

== system LoFT_Example3/FOWT System/Subsystem7/switch 3 ==
  note: communictation failure occurs when switch ==0
  In1 : Inport
  Constant : Constant  Value=0
  Mux : Mux  Inputs=2
  Out1 : Outport
  wires:
  Constant/1 -> Mux/2
  In1/1 -> Mux/1
  Mux/1 -> Out1/1

== system LoFT_Example3/FOWT System/Subsystem7/switch 4 ==
  note: communictation failure occurs when switch ==0
  In1 : Inport
  Constant : Constant  Value=0
  Mux : Mux  Inputs=2
  Out1 : Outport
  wires:
  Mux/1 -> Out1/1
  In1/1 -> Mux/1
  Constant/1 -> Mux/2

== system LoFT_Example3/FOWT System/Subsystem7/switch 5 ==
  note: communictation failure occurs when switch ==0
  In1 : Inport
  Constant : Constant  Value=0
  Mux : Mux  Inputs=2
  Out1 : Outport
  wires:
  Constant/1 -> Mux/2
  In1/1 -> Mux/1
  Mux/1 -> Out1/1

== system LoFT_Example3/FOWT System/Subsystem7/switch 6 ==
  note: communictation failure occurs when switch ==0
  In1 : Inport
  Constant : Constant  Value=0
  Mux : Mux  Inputs=2
  Out1 : Outport
  wires:
  Mux/1 -> Out1/1
  In1/1 -> Mux/1
  Constant/1 -> Mux/2

== system LoFT_Example3/FOWT System/Subsystem7/switch 7 ==
  note: communictation failure occurs when switch ==0
  In1 : Inport
  Constant : Constant  Value=0
  Mux : Mux  Inputs=2
  Out1 : Outport
  wires:
  Constant/1 -> Mux/2
  In1/1 -> Mux/1
  Mux/1 -> Out1/1

== system LoFT_Example3/FOWT System/Subsystem7/switch 8 ==
  note: communictation failure occurs when switch ==0
  In1 : Inport
  Constant : Constant  Value=0
  Mux : Mux  Inputs=2
  Out1 : Outport
  wires:
  Constant/1 -> Mux/2
  In1/1 -> Mux/1
  Mux/1 -> Out1/1

== system LoFT_Example3/FOWT System/Subsystem7/switch 9 ==
  note: communictation failure occurs when switch ==0
  In1 : Inport
  Constant : Constant  Value=0
  Mux : Mux  Inputs=2
  Out1 : Outport
  wires:
  Constant/1 -> Mux/2
  In1/1 -> Mux/1
  Mux/1 -> Out1/1

== system LoFT_Example3/FOWT System/Subsystem7/wave series 1 ==
  1-D Lookup Table : Lookup_n-D  NumberOfTableDimensions=1  BreakpointsForDimension1=LoFT.Hydro.waveforces.time  Table=squeeze(LoFT.Hydro.waveforces.force(1,1,:))  InternalRulePriority=Speed  RndMeth=Simplest
  1-D Lookup Table1 : Lookup_n-D  NumberOfTableDimensions=1  BreakpointsForDimension1=LoFT.Hydro.waveforces.time  Table=squeeze(LoFT.Hydro.waveforces.force(1,2,:))  InternalRulePriority=Speed  RndMeth=Simplest
  1-D Lookup Table2 : Lookup_n-D  NumberOfTableDimensions=1  BreakpointsForDimension1=LoFT.Hydro.waveforces.time  Table=squeeze(LoFT.Hydro.waveforces.force(1,3,:))  InternalRulePriority=Speed  RndMeth=Simplest
  Clock1 : Clock
  Clock2 : Clock
  Clock3 : Clock
  Vector Concatenate1 : Concatenate  NumInputs=3
  Out1 : Outport
  wires:
  Vector Concatenate1/1 -> Out1/1
  Clock2/1 -> 1-D Lookup Table1/1
  1-D Lookup Table/1 -> Vector Concatenate1/1
  Clock3/1 -> 1-D Lookup Table2/1
  Clock1/1 -> 1-D Lookup Table/1
  1-D Lookup Table1/1 -> Vector Concatenate1/2
  1-D Lookup Table2/1 -> Vector Concatenate1/3

== system LoFT_Example3/FOWT System/Subsystem7/wave series 10 ==
  1-D Lookup Table : Lookup_n-D  NumberOfTableDimensions=1  BreakpointsForDimension1=LoFT.Hydro.waveforces.time + 10  Table=squeeze(LoFT.Hydro.waveforces.force(1,1,:))  InternalRulePriority=Speed  RndMeth=Simplest
  1-D Lookup Table1 : Lookup_n-D  NumberOfTableDimensions=1  BreakpointsForDimension1=LoFT.Hydro.waveforces.time + 10  Table=squeeze(LoFT.Hydro.waveforces.force(1,2,:))  InternalRulePriority=Speed  RndMeth=Simplest
  1-D Lookup Table2 : Lookup_n-D  NumberOfTableDimensions=1  BreakpointsForDimension1=LoFT.Hydro.waveforces.time + 10  Table=squeeze(LoFT.Hydro.waveforces.force(1,3,:))  InternalRulePriority=Speed  RndMeth=Simplest
  Clock1 : Clock
  Clock2 : Clock
  Clock3 : Clock
  Vector Concatenate1 : Concatenate  NumInputs=3
  Out1 : Outport
  wires:
  1-D Lookup Table2/1 -> Vector Concatenate1/3
  1-D Lookup Table1/1 -> Vector Concatenate1/2
  Clock1/1 -> 1-D Lookup Table/1
  Clock3/1 -> 1-D Lookup Table2/1
  1-D Lookup Table/1 -> Vector Concatenate1/1
  Clock2/1 -> 1-D Lookup Table1/1
  Vector Concatenate1/1 -> Out1/1

== system LoFT_Example3/FOWT System/Subsystem7/wave series 2 ==
  1-D Lookup Table : Lookup_n-D  NumberOfTableDimensions=1  BreakpointsForDimension1=LoFT.Hydro.waveforces.time + 5  Table=squeeze(LoFT.Hydro.waveforces.force(1,1,:))  InternalRulePriority=Speed  RndMeth=Simplest
  1-D Lookup Table1 : Lookup_n-D  NumberOfTableDimensions=1  BreakpointsForDimension1=LoFT.Hydro.waveforces.time + 5  Table=squeeze(LoFT.Hydro.waveforces.force(1,2,:))  InternalRulePriority=Speed  RndMeth=Simplest
  1-D Lookup Table2 : Lookup_n-D  NumberOfTableDimensions=1  BreakpointsForDimension1=LoFT.Hydro.waveforces.time + 5  Table=squeeze(LoFT.Hydro.waveforces.force(1,3,:))  InternalRulePriority=Speed  RndMeth=Simplest
  Clock1 : Clock
  Clock2 : Clock
  Clock3 : Clock
  Vector Concatenate1 : Concatenate  NumInputs=3
  Out1 : Outport
  wires:
  1-D Lookup Table2/1 -> Vector Concatenate1/3
  1-D Lookup Table1/1 -> Vector Concatenate1/2
  Clock1/1 -> 1-D Lookup Table/1
  Clock3/1 -> 1-D Lookup Table2/1
  1-D Lookup Table/1 -> Vector Concatenate1/1
  Clock2/1 -> 1-D Lookup Table1/1
  Vector Concatenate1/1 -> Out1/1

== system LoFT_Example3/FOWT System/Subsystem7/wave series 3 ==
  1-D Lookup Table : Lookup_n-D  NumberOfTableDimensions=1  BreakpointsForDimension1=LoFT.Hydro.waveforces.time + 10  Table=squeeze(LoFT.Hydro.waveforces.force(1,1,:))  InternalRulePriority=Speed  RndMeth=Simplest
  1-D Lookup Table1 : Lookup_n-D  NumberOfTableDimensions=1  BreakpointsForDimension1=LoFT.Hydro.waveforces.time + 10  Table=squeeze(LoFT.Hydro.waveforces.force(1,2,:))  InternalRulePriority=Speed  RndMeth=Simplest
  1-D Lookup Table2 : Lookup_n-D  NumberOfTableDimensions=1  BreakpointsForDimension1=LoFT.Hydro.waveforces.time + 10  Table=squeeze(LoFT.Hydro.waveforces.force(1,3,:))  InternalRulePriority=Speed  RndMeth=Simplest
  Clock1 : Clock
  Clock2 : Clock
  Clock3 : Clock
  Vector Concatenate1 : Concatenate  NumInputs=3
  Out1 : Outport
  wires:
  Vector Concatenate1/1 -> Out1/1
  Clock2/1 -> 1-D Lookup Table1/1
  1-D Lookup Table/1 -> Vector Concatenate1/1
  Clock3/1 -> 1-D Lookup Table2/1
  Clock1/1 -> 1-D Lookup Table/1
  1-D Lookup Table1/1 -> Vector Concatenate1/2
  1-D Lookup Table2/1 -> Vector Concatenate1/3

== system LoFT_Example3/FOWT System/Subsystem7/wave series 4 ==
  1-D Lookup Table : Lookup_n-D  NumberOfTableDimensions=1  BreakpointsForDimension1=LoFT.Hydro.waveforces.time+15  Table=squeeze(LoFT.Hydro.waveforces.force(1,1,:))  InternalRulePriority=Speed  RndMeth=Simplest
  1-D Lookup Table1 : Lookup_n-D  NumberOfTableDimensions=1  BreakpointsForDimension1=LoFT.Hydro.waveforces.time+15  Table=squeeze(LoFT.Hydro.waveforces.force(1,2,:))  InternalRulePriority=Speed  RndMeth=Simplest
  1-D Lookup Table2 : Lookup_n-D  NumberOfTableDimensions=1  BreakpointsForDimension1=LoFT.Hydro.waveforces.time+15  Table=squeeze(LoFT.Hydro.waveforces.force(1,3,:))  InternalRulePriority=Speed  RndMeth=Simplest
  Clock1 : Clock
  Clock2 : Clock
  Clock3 : Clock
  Vector Concatenate1 : Concatenate  NumInputs=3
  Out1 : Outport
  wires:
  1-D Lookup Table2/1 -> Vector Concatenate1/3
  1-D Lookup Table1/1 -> Vector Concatenate1/2
  Clock1/1 -> 1-D Lookup Table/1
  Clock3/1 -> 1-D Lookup Table2/1
  1-D Lookup Table/1 -> Vector Concatenate1/1
  Clock2/1 -> 1-D Lookup Table1/1
  Vector Concatenate1/1 -> Out1/1

== system LoFT_Example3/FOWT System/Subsystem7/wave series 5 ==
  1-D Lookup Table : Lookup_n-D  NumberOfTableDimensions=1  BreakpointsForDimension1=LoFT.Hydro.waveforces.time+20  Table=squeeze(LoFT.Hydro.waveforces.force(1,1,:))  InternalRulePriority=Speed  RndMeth=Simplest
  1-D Lookup Table1 : Lookup_n-D  NumberOfTableDimensions=1  BreakpointsForDimension1=LoFT.Hydro.waveforces.time+20  Table=squeeze(LoFT.Hydro.waveforces.force(1,2,:))  InternalRulePriority=Speed  RndMeth=Simplest
  1-D Lookup Table2 : Lookup_n-D  NumberOfTableDimensions=1  BreakpointsForDimension1=LoFT.Hydro.waveforces.time+20  Table=squeeze(LoFT.Hydro.waveforces.force(1,3,:))  InternalRulePriority=Speed  RndMeth=Simplest
  Clock1 : Clock
  Clock2 : Clock
  Clock3 : Clock
  Vector Concatenate1 : Concatenate  NumInputs=3
  Out1 : Outport
  wires:
  Vector Concatenate1/1 -> Out1/1
  Clock2/1 -> 1-D Lookup Table1/1
  1-D Lookup Table/1 -> Vector Concatenate1/1
  Clock3/1 -> 1-D Lookup Table2/1
  Clock1/1 -> 1-D Lookup Table/1
  1-D Lookup Table1/1 -> Vector Concatenate1/2
  1-D Lookup Table2/1 -> Vector Concatenate1/3

== system LoFT_Example3/FOWT System/Subsystem7/wave series 6 ==
  1-D Lookup Table : Lookup_n-D  NumberOfTableDimensions=1  BreakpointsForDimension1=LoFT.Hydro.waveforces.time + 10  Table=squeeze(LoFT.Hydro.waveforces.force(1,1,:))  InternalRulePriority=Speed  RndMeth=Simplest
  1-D Lookup Table1 : Lookup_n-D  NumberOfTableDimensions=1  BreakpointsForDimension1=LoFT.Hydro.waveforces.time + 10  Table=squeeze(LoFT.Hydro.waveforces.force(1,2,:))  InternalRulePriority=Speed  RndMeth=Simplest
  1-D Lookup Table2 : Lookup_n-D  NumberOfTableDimensions=1  BreakpointsForDimension1=LoFT.Hydro.waveforces.time + 10  Table=squeeze(LoFT.Hydro.waveforces.force(1,3,:))  InternalRulePriority=Speed  RndMeth=Simplest
  Clock1 : Clock
  Clock2 : Clock
  Clock3 : Clock
  Vector Concatenate1 : Concatenate  NumInputs=3
  Out1 : Outport
  wires:
  1-D Lookup Table2/1 -> Vector Concatenate1/3
  1-D Lookup Table1/1 -> Vector Concatenate1/2
  Clock1/1 -> 1-D Lookup Table/1
  Clock3/1 -> 1-D Lookup Table2/1
  1-D Lookup Table/1 -> Vector Concatenate1/1
  Clock2/1 -> 1-D Lookup Table1/1
  Vector Concatenate1/1 -> Out1/1

== system LoFT_Example3/FOWT System/Subsystem7/wave series 7 ==
  1-D Lookup Table : Lookup_n-D  NumberOfTableDimensions=1  BreakpointsForDimension1=LoFT.Hydro.waveforces.time + 10  Table=squeeze(LoFT.Hydro.waveforces.force(1,1,:))  InternalRulePriority=Speed  RndMeth=Simplest
  1-D Lookup Table1 : Lookup_n-D  NumberOfTableDimensions=1  BreakpointsForDimension1=LoFT.Hydro.waveforces.time + 10  Table=squeeze(LoFT.Hydro.waveforces.force(1,2,:))  InternalRulePriority=Speed  RndMeth=Simplest
  1-D Lookup Table2 : Lookup_n-D  NumberOfTableDimensions=1  BreakpointsForDimension1=LoFT.Hydro.waveforces.time + 10  Table=squeeze(LoFT.Hydro.waveforces.force(1,3,:))  InternalRulePriority=Speed  RndMeth=Simplest
  Clock1 : Clock
  Clock2 : Clock
  Clock3 : Clock
  Vector Concatenate1 : Concatenate  NumInputs=3
  Out1 : Outport
  wires:
  Vector Concatenate1/1 -> Out1/1
  Clock2/1 -> 1-D Lookup Table1/1
  1-D Lookup Table/1 -> Vector Concatenate1/1
  Clock3/1 -> 1-D Lookup Table2/1
  Clock1/1 -> 1-D Lookup Table/1
  1-D Lookup Table1/1 -> Vector Concatenate1/2
  1-D Lookup Table2/1 -> Vector Concatenate1/3

== system LoFT_Example3/FOWT System/Subsystem7/wave series 8 ==
  1-D Lookup Table : Lookup_n-D  NumberOfTableDimensions=1  BreakpointsForDimension1=LoFT.Hydro.waveforces.time + 10  Table=squeeze(LoFT.Hydro.waveforces.force(1,1,:))  InternalRulePriority=Speed  RndMeth=Simplest
  1-D Lookup Table1 : Lookup_n-D  NumberOfTableDimensions=1  BreakpointsForDimension1=LoFT.Hydro.waveforces.time + 10  Table=squeeze(LoFT.Hydro.waveforces.force(1,2,:))  InternalRulePriority=Speed  RndMeth=Simplest
  1-D Lookup Table2 : Lookup_n-D  NumberOfTableDimensions=1  BreakpointsForDimension1=LoFT.Hydro.waveforces.time + 10  Table=squeeze(LoFT.Hydro.waveforces.force(1,3,:))  InternalRulePriority=Speed  RndMeth=Simplest
  Clock1 : Clock
  Clock2 : Clock
  Clock3 : Clock
  Vector Concatenate1 : Concatenate  NumInputs=3
  Out1 : Outport
  wires:
  1-D Lookup Table2/1 -> Vector Concatenate1/3
  1-D Lookup Table1/1 -> Vector Concatenate1/2
  Clock1/1 -> 1-D Lookup Table/1
  Clock3/1 -> 1-D Lookup Table2/1
  1-D Lookup Table/1 -> Vector Concatenate1/1
  Clock2/1 -> 1-D Lookup Table1/1
  Vector Concatenate1/1 -> Out1/1
